simulink model "simulacao"  (R2023b)
settings: Solver=ode4  StartTime=0.0  StopTime=80  FixedStep=0.001  RelTol=1e-3
InitFcn:
  | alpha = 20.70;
  | beta =  1.27;
  | gamma = 0.53;
undefined symbols (not defined in the file or in its folder): sigbuilder_block
libraries: simulink_extras x2, cstextras x1
settings Model: SimulationMode=accelerator  Creator=colom  LastModifiedBy=Paulo
settings SolverCC: AlgebraicLoopSolver=TrustRegion  AutoInsertRateTranBlk=on
settings OptimizationCC: LifeSpan=inf
settings DebuggingCC: SFExecutionAtInitializationDiag=none  ArithmeticOperatorsInVariantConditions=warning
settings HardwareCC: ProdBitPerSizeT=32  ProdBitPerPtrDiffT=32  ProdWordSize=32  ProdHWDeviceType=Specified
settings ModelReferenceCC: EnableRefExpFcnMdlSchedulingChecks=on
settings SFSimCC: CustomCodeUndefinedFunction=UseInterfaceOnly
settings CodeAppCC: StateflowObjectComments=on

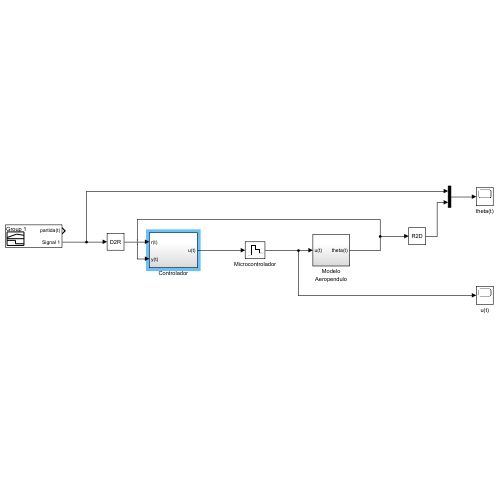
[thumbnail: Simulink's stored preview of the top-level diagram]
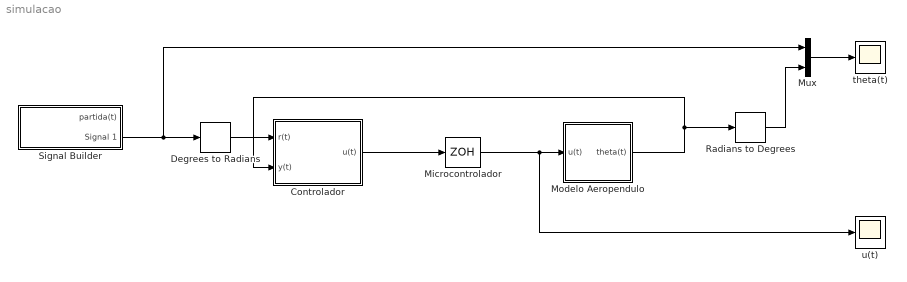
== system simulacao ==
  Controlador : Subsystem
  Degrees to Radians : simulink_extras/Transformations/Degrees to Radians
  Microcontrolador : ZeroOrderHold  SampleTime=0.020
  Modelo Aeropendulo : Subsystem
  Mux : Mux  Inputs=2
  Radians to Degrees : simulink_extras/Transformations/Radians to Degrees
  Signal Builder : Subsystem  Tag=STV Subsys  LoadFcn=sigbuilder_block('load');  StartFcn=sigbuilder_block('start');  StopFcn=sigbuilder_block('stop');  ClipboardFcn=sigbuilder_block('clipboard');  mask(Sigbuilder block){tuvar=[0:10]}
      mask help: Simulink:masks:SigbuilderBlock_MD
      mask init:
      | if ~strcmp(get_param(bdroot(gcbh),'SimulationStatus'),'stopped') tuvar = sigbuilder_block('maskInit'); end
      settings: CopyFcn=sigbuilder_block('copy');  DeleteFcn=sigbuilder_block('delete');  ModelCloseFcn=sigbuilder_block('modelClose');  PreSaveFcn=sigbuilder_block('preSave');  PauseFcn=sigbuilder_block('pause');  ContinueFcn=sigbuilder_block('continue');  NameChangeFcn=sigbuilder_block('namechange');  OpenFcn=sigbuilder_block('open',[5.4 36 1141.2 516.6 ]);  CloseFcn=sigbuilder_block('close');
      mask Display: plot(0, 0, 100, 100,[2, 2, 32, 32, 2], [68, 8, 8, 68, 68],[32, 2], [38, 38], [32, 19, 2],[53, 60, 44], [32, 17, 17, 2],[16, 16, 31, 31]);txt = getActiveGroup(gcbh);text(2, 100, txt,'verticalAlignment', 'top');
  theta(t) : Scope
  u(t) : Scope
  wires:
  Microcontrolador/1 -> Modelo Aeropendulo/1(u(t)), u(t)/1
  Modelo Aeropendulo/1(theta(t)) -> Controlador/2(y(t)), Radians to Degrees/1
  Mux/1 -> theta(t)/1
  Radians to Degrees/1 -> Mux/2
  Signal Builder/2(Signal 1) -> Mux/1, Degrees to Radians/1
  Degrees to Radians/1 -> Controlador/1(r(t))
  Controlador/1(u(t)) -> Microcontrolador/1

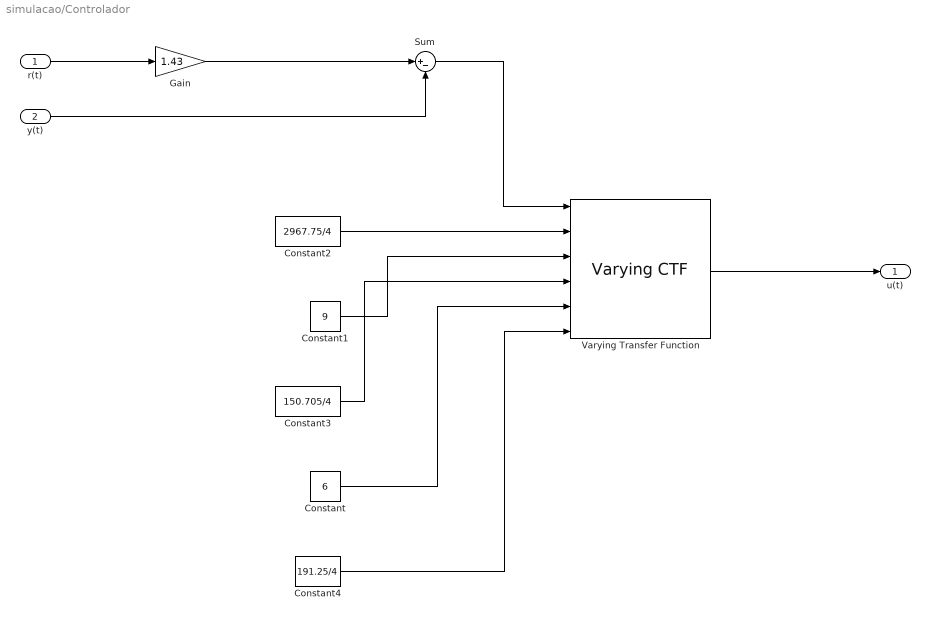
== system simulacao/Controlador ==
  r(t) : Inport
  y(t) : Inport  Port=2
  Constant : Constant  Value=6
  Constant1 : Constant  Value=9
  Constant2 : Constant  Value=2967.75/4
  Constant3 : Constant  Value=150.705/4
  Constant4 : Constant  Value=191.25/4
  Gain : Gain  Gain=1.43
  Sum : Sum  Inputs=|+-
  Varying Transfer Function : cstextras/Varying CTF  N=2
  u(t) : Outport  VectorParamsAs1DForOutWhenUnconnected=off
  wires:
  Constant3/1 -> Varying Transfer Function/4
  Constant1/1 -> Varying Transfer Function/3
  Sum/1 -> Varying Transfer Function/1
  y(t)/1 -> Sum/2
  Varying Transfer Function/1 -> u(t)/1
  Gain/1 -> Sum/1
  r(t)/1 -> Gain/1
  Constant2/1 -> Varying Transfer Function/2
  Constant4/1 -> Varying Transfer Function/6
  Constant/1 -> Varying Transfer Function/5

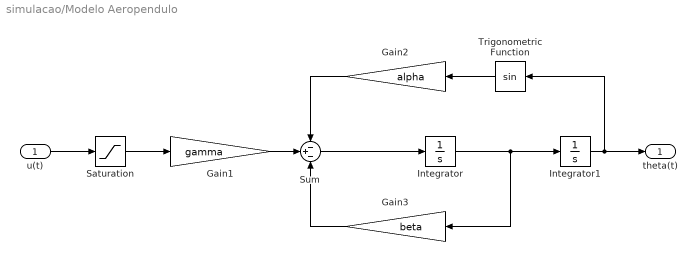
== system simulacao/Modelo Aeropendulo ==
  u(t) : Inport
  Gain1 : Gain  Gain=gamma
  Gain2 : Gain  Gain=alpha
  Gain3 : Gain  Gain=beta
  Integrator : Integrator
  Integrator1 : Integrator
  Saturation : Saturate  UpperLimit=100  LowerLimit=0
  Sum : Sum  Inputs=-+-
  Trigonometric Function : Trigonometry
  theta(t) : Outport  VectorParamsAs1DForOutWhenUnconnected=off
  wires:
  Gain3/1 -> Sum/3
  u(t)/1 -> Saturation/1
  Integrator1/1 -> theta(t)/1, Trigonometric Function/1
  Trigonometric Function/1 -> Gain2/1
  Gain2/1 -> Sum/1
  Integrator/1 -> Gain3/1, Integrator1/1
  Sum/1 -> Integrator/1
  Gain1/1 -> Sum/2
  Saturation/1 -> Gain1/1

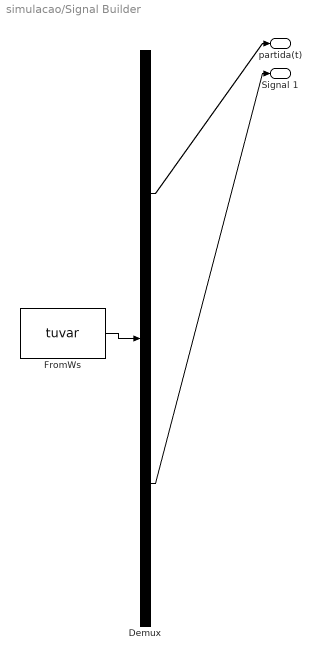
== system simulacao/Signal Builder ==
  Demux : Demux  Tag=STV Demux  Outputs=2
      settings: DisplayOption=none
  FromWs : FromWorkspace  Tag=STV FromWs  VariableName=tuvar
      SigBuilderData=|
      | common.afterFinalStr = 'Extrapolate'
      | common.sampleTime = 0
      | dataSet.timeRange = [0 80]
      | dataSet.name = 'Group 1'
      | sbobj.Groups.Name = 'Group 1'
      | sbobj.Groups.Signals(1).Name = 'partida(t)'
      | sbobj.Groups.Signals(1).XData = [0 0.5 0.5 2.5 2.5 6.5 6.5 10 10 15 16 17 18 19 80]
      | sbobj.Groups.Signals(1).YData = [0 0 2000 2000 2 0 1040 1040 4 0 0 0 0 0 0]
      | sbobj.Groups.Signals(2).Name = 'Signal 1'
      | sbobj.Groups.Signals(2).XData = [0 10 15 20 30 30 36 39 47 52 72 73 74 75 76 77 78 79 80]
      | sbobj.Groups.Signals(2).YData = [0 0 15 30 30 35 35 35 35 35 0 0 0 0 0 0 0 0 0]
      | sbobj.Groups.TimeRange = [0 80]
  partida(t) : Outport  Tag=STV Outport  VectorParamsAs1DForOutWhenUnconnected=off
  Signal 1 : Outport  Tag=STV Outport  Port=2  VectorParamsAs1DForOutWhenUnconnected=off
  wires:
  FromWs/1 -> Demux/1
  Demux/1 -> partida(t)/1
  Demux/2 -> Signal 1/1
